simulink model "Problem_5_sdomain"  (R2020a)
settings: Solver=VariableStepAuto  StartTime=0.0  StopTime=inf  RelTol=1e-3
model workspace (MAT data in the model file):
  C = 0.005
  R = 10
settings Model: Creator=Shubham Singh Rathor  LastModifiedBy=Shubham Singh Rathor

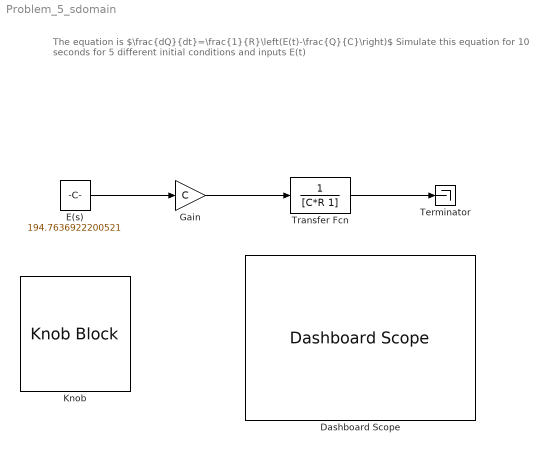
== system Problem_5_sdomain ==
  note: The equation is
      | $\frac{dQ}{dt}=\frac{1}{R}\left(E(t)-\frac{Q}{C}\right)$
      | Simulate this equation for 10 seconds for 5 different initial conditions and inputs E(t)
  Dashboard Scope : DashboardScope
  E(s) : Constant  Value=194.7636922200521
  Gain : Gain  Gain=C
  Knob : KnobBlock  LabelPosition=Bottom  ScaleMax=200
  Terminator : Terminator
  Transfer Fcn : TransferFcn  Denominator=[C*R 1]
  wires:
  E(s)/1 -> Gain/1
  Gain/1 -> Transfer Fcn/1
  Transfer Fcn/1 -> Terminator/1
